simulink model "Pedal_Interpretation_exe_gr"  (Simulink 7.0)
settings: Solver=ode4  StartTime=0.0  StopTime=88  FixedStep=0.01  RelTol=1e-3
InitFcn:
  | PedalInterp_para
values from neighbouring files (symbols this model uses):
  ped_min = 5    [PedalInterp_para.m]
  T_max_Brake = 4000    [PedalInterp_para.m]
  TI = 0    [PAS_callback.m]
undefined symbols (not defined in the file or in its folder): fzgbib, m_ab_100pro, m_ab_70pro, PedalInterpretation, v_bereich
libraries: simulink x320
(part 3 of 23)

== system Pedal_Interpretation_exe_gr/Test Specification for PI/SR-PI-02.2 Acceleration pedal interpretation/v = const & phi_Acc = const ==
  InOut Bus : Inport  OutDataType=sfix(16)  OutScaling=2^0
  Bus Selector : BusSelector  OutputSignals=Inputs.v_Fzg,Inputs.signal2.phi_Acc
  Constant : Constant  OutDataType=sfix(16)  OutScaling=2^0
  Constant1 : Constant  OutDataType=sfix(16)  OutScaling=2^0
  Detect constant : Subsystem  TreatAsAtomicUnit=on  mask(Feature extraction block){RT=1}
      mask prompts: RT "Relative tolerance in %"
      mask help: Detect if the signal value is constant (using the last two signal values) allowing for a user-defined relative deviation
      mask CallbackString:
      | if or( (str2double(get_param(gcb,'RT')) < 0), (str2double(get_param(gcb,'RT')) > 100))
      |     error(['Relative tolerance value (' get_param(gcb,'RT') ') out of range. Please give a value between 0 and 100.']);
      | else
      |     set_param([gcb '/Relative tolerance/Relative Tolerance'],'Value',get_param(gcb,'RT'));
      | end
  Detect constant1 : Subsystem  TreatAsAtomicUnit=on  mask(Feature extraction block){RT=1}
      mask prompts: RT "Relative tolerance in %"
      mask help: Detect if the signal value is constant (using the last two signal values) allowing for a user-defined relative deviation
      mask CallbackString:
      | if or( (str2double(get_param(gcb,'RT')) < 0), (str2double(get_param(gcb,'RT')) > 100))
      |     error(['Relative tolerance value (' get_param(gcb,'RT') ') out of range. Please give a value between 0 and 100.']);
      | else
      |     set_param([gcb '/Relative tolerance/Relative Tolerance'],'Value',get_param(gcb,'RT'));
      | end
  PS : Subsystem  mask(Feature layer: preconditions synchronization){NoTI=2, NoTDD=0, NoTID=0, TIdel=[2  2], TDDdel=[]}
      mask prompts: NoTI "Time-independent features identifiable with or without a delay (TI)"; NoTDD "Triggered features identifiable with determinate delay or without a delay (TDD)"; NoTID "Triggered features identifiable with indeterminate delay (TID)"; TIdel "Time-independent features delays (in time steps). E.g. [0 1 0] for 3 features"; TDDdel "Triggered features delays (in time steps). E.g. [0 0] for 2 features"
      mask help: Use this block for synchronizing the precondition features. For changing the block inputs, use the parameters below. The output must be used for assertions activation.
      mask init:
      | PS_init(gcb);
      mask StyleString: popup(0|1|2|3|4|5|6|7|8|9),popup(0|1|2|3|4|5|6|7|8|9),popup(0|1|2|3|4|5|6|7|8|9),edit,edit
      mask CallbackString:
      | PSTI_callback(gcb);|PSTDD_callback(gcb);|PSTID_callback(gcb);|NoTI = str2double(get_param(gcb,'NoTI'));
      | TIdel = str2num(get_param(gcb,'TIdel'));
      | if NoTI ~= length(TIdel) && NoTI ~= 0
      |     error(['The number of delays entered (' num2str(length(TIdel)) ') does not correspond to the above specified number of time-independent features (' num2str(NoTI) ').']);
      | end|NoTDD = str2double(get_param(gcb,'NoTDD'));
      | TDDdel = str2num(get_param(gcb,'TDDdel'));
      | if NoTDD ~= length(TDDdel) && NoTDD ~= 0
      |     error(['The number of delays entered (' num2str(length(TDDdel)) ') does not correspond to the above specified number of triggered features with constant delay (' num2str(NoTDD) ').']);
      | end
  Range - Gap Relative tolerance Precond : Subsystem  mask(Range - Gap Relative Tolerance){GorR=Range, RelativeTolerance=0}
      mask prompts: GorR "Use range or gap"; RelativeTolerance "Relative Tolerance in Percent"
      mask help: Check that a signal stays inside a range or outside a gap around a reference signal. Specify the range or the gap relative to the reference signal.
      mask init: same as Pedal_Interpretation_exe_gr/Test Specification for PI/SR-PI-01.1 Brake Pedal recognition/BrakePedal == 0/Range - Gap Relative tolerance Ass
      mask StyleString: popup(Range|Gap  ),edit
      mask Display:
      | port_label('output',1,'A');
      | port_label('input',1,'Sig');
      | port_label('input',2,'Ref');
      | text(0.35,0.5,[num2str(RelativeTolerance) '%']);
      | text(0.05,0.5,helpVariable2);
  Range - Gap Relative tolerance Precond1 : Subsystem  mask(Range - Gap Relative Tolerance){GorR=Range, RelativeTolerance=0}
      mask prompts: GorR "Use range or gap"; RelativeTolerance "Relative Tolerance in Percent"
      mask help: Check that a signal stays inside a range or outside a gap around a reference signal. Specify the range or the gap relative to the reference signal.
      mask init: same as Pedal_Interpretation_exe_gr/Test Specification for PI/SR-PI-01.1 Brake Pedal recognition/BrakePedal == 0/Range - Gap Relative tolerance Ass
      mask StyleString: popup(Range|Gap  ),edit
      mask Display:
      | port_label('output',1,'A');
      | port_label('input',1,'Sig');
      | port_label('input',2,'Ref');
      | text(0.35,0.5,[num2str(RelativeTolerance) '%']);
      | text(0.05,0.5,helpVariable2);
  Activate : Outport  OutDataType=sfix(16)  OutScaling=2^0
  wires:
  InOut Bus/1 -> Bus Selector/1
  Bus Selector/1 -> Detect constant/1(Signal)  "<v_Fzg>"
  Bus Selector/2 -> Detect constant1/1(Signal)  "<phi_Acc>"
  PS/1(Precond) -> Activate/1
  Detect constant/1(Constant) -> Range - Gap Relative tolerance Precond/1(Signal)
  Constant/1 -> Range - Gap Relative tolerance Precond/2(Reference)
  Detect constant1/1(Constant) -> Range - Gap Relative tolerance Precond1/1(Signal)
  Constant1/1 -> Range - Gap Relative tolerance Precond1/2(Reference)
  Range - Gap Relative tolerance Precond/1(Activate) -> PS/1(A TI1)
  Range - Gap Relative tolerance Precond1/1(Activate) -> PS/2(A TI2)

== system Pedal_Interpretation_exe_gr/Test Specification for PI/SR-PI-02.2 Acceleration pedal interpretation/v = const & phi_Acc decreases & T_des_Drive < 0 ==
  InOut Bus : Inport  OutDataType=sfix(16)  OutScaling=2^0
  Bound Precond : Subsystem  mask(Bound){cm=<}
      mask prompts: cm "Comparison method:"
      mask help:
      | Compare a signal with a reference using the specified comparison method.
      |
      | For '==' or '~=' use "Range - Gap"
      mask init:
      | bp = get_param(gcbh,'Parent');
      | bn = get_param(gcbh,'Name');
      | set_param([bp '/' bn '/RelOp'],'Operator',get_param(gcbh,'cm'));
      mask StyleString: popup(>|>=|<=|<)
      mask Display:
      | port_label('output', 1, 'A');
      | port_label('input', 1, 'Sig');
      | port_label('input', 2, 'Ref');
      | text(0.05,0.5,get_param(get_param([get_param(gcb,'Parent') '/' get_param(gcb,'Name') '/RelOp'],'handle'),'Operator'));
  Bus Selector : BusSelector  OutputSignals=Inputs.v_Fzg,Inputs.signal2.phi_Acc,Outputs.signal1.T_des_Drive
  Constant : Constant  OutDataType=sfix(16)  OutScaling=2^0
  Constant1 : Constant  OutDataType=sfix(16)  OutScaling=2^0
  Constant2 : Constant  Value=0  OutDataType=sfix(16)  OutScaling=2^0
  Detect constant : Subsystem  TreatAsAtomicUnit=on  mask(Feature extraction block){RT=0}
      mask prompts: RT "Relative tolerance in %"
      mask help: Detect if the signal value is constant (using the last two signal values) allowing for a user-defined relative deviation
      mask CallbackString:
      | if or( (str2double(get_param(gcb,'RT')) < 0), (str2double(get_param(gcb,'RT')) > 100))
      |     error(['Relative tolerance value (' get_param(gcb,'RT') ') out of range. Please give a value between 0 and 100.']);
      | else
      |     set_param([gcb '/Relative tolerance/Relative Tolerance'],'Value',get_param(gcb,'RT'));
      | end
  Detect decrease : Subsystem  TreatAsAtomicUnit=on  mask(Detect increase){Param=0}
      mask prompts: Param "Mask Parameter 1:"
  PS : Subsystem  mask(Feature layer: preconditions synchronization){NoTI=3, NoTDD=0, NoTID=0, TIdel=[2  2  2], TDDdel=[]}
      mask prompts: NoTI "Time-independent features identifiable with or without a delay (TI)"; NoTDD "Triggered features identifiable with determinate delay or without a delay (TDD)"; NoTID "Triggered features identifiable with indeterminate delay (TID)"; TIdel "Time-independent features delays (in time steps). E.g. [0 1 0] for 3 features"; TDDdel "Triggered features delays (in time steps). E.g. [0 0] for 2 features"
      mask help: Use this block for synchronizing the precondition features. For changing the block inputs, use the parameters below. The output must be used for assertions activation.
      mask init:
      | PS_init(gcb);
      mask StyleString: popup(0|1|2|3|4|5|6|7|8|9),popup(0|1|2|3|4|5|6|7|8|9),popup(0|1|2|3|4|5|6|7|8|9),edit,edit
      mask CallbackString:
      | PSTI_callback(gcb);|PSTDD_callback(gcb);|PSTID_callback(gcb);|NoTI = str2double(get_param(gcb,'NoTI'));
      | TIdel = str2num(get_param(gcb,'TIdel'));
      | if NoTI ~= length(TIdel) && NoTI ~= 0
      |     error(['The number of delays entered (' num2str(length(TIdel)) ') does not correspond to the above specified number of time-independent features (' num2str(NoTI) ').']);
      | end|NoTDD = str2double(get_param(gcb,'NoTDD'));
      | TDDdel = str2num(get_param(gcb,'TDDdel'));
      | if NoTDD ~= length(TDDdel) && NoTDD ~= 0
      |     error(['The number of delays entered (' num2str(length(TDDdel)) ') does not correspond to the above specified number of triggered features with constant delay (' num2str(NoTDD) ').']);
      | end
  Range - Gap Relative tolerance Precond : Subsystem  mask(Range - Gap Relative Tolerance){GorR=Range, RelativeTolerance=0}
      mask prompts: GorR "Use range or gap"; RelativeTolerance "Relative Tolerance in Percent"
      mask help: Check that a signal stays inside a range or outside a gap around a reference signal. Specify the range or the gap relative to the reference signal.
      mask init: same as Pedal_Interpretation_exe_gr/Test Specification for PI/SR-PI-01.1 Brake Pedal recognition/BrakePedal == 0/Range - Gap Relative tolerance Ass
      mask StyleString: popup(Range|Gap  ),edit
      mask Display:
      | port_label('output',1,'A');
      | port_label('input',1,'Sig');
      | port_label('input',2,'Ref');
      | text(0.35,0.5,[num2str(RelativeTolerance) '%']);
      | text(0.05,0.5,helpVariable2);
  Range - Gap Relative tolerance Precond1 : Subsystem  mask(Range - Gap Relative Tolerance){GorR=Range, RelativeTolerance=0}
      mask prompts: GorR "Use range or gap"; RelativeTolerance "Relative Tolerance in Percent"
      mask help: Check that a signal stays inside a range or outside a gap around a reference signal. Specify the range or the gap relative to the reference signal.
      mask init: same as Pedal_Interpretation_exe_gr/Test Specification for PI/SR-PI-01.1 Brake Pedal recognition/BrakePedal == 0/Range - Gap Relative tolerance Ass
      mask StyleString: popup(Range|Gap  ),edit
      mask Display:
      | port_label('output',1,'A');
      | port_label('input',1,'Sig');
      | port_label('input',2,'Ref');
      | text(0.35,0.5,[num2str(RelativeTolerance) '%']);
      | text(0.05,0.5,helpVariable2);
  Scope1 : Scope  NumInputPorts=4
      settings: YMin=-5~-5~-5~-5  YMax=5~5~5~5  SaveName=ScopeData10  MaxDataPoints=11115000
  Activate : Outport  OutDataType=sfix(16)  OutScaling=2^0
  wires:
  PS/1(Precond) -> Activate/1
  InOut Bus/1 -> Bus Selector/1
  Bus Selector/1 -> Detect constant/1(Signal)  "<v_Fzg>"
  Bus Selector/2 -> Detect decrease/1(Signal)  "<phi_Acc>"
  Constant/1 -> Range - Gap Relative tolerance Precond/2(Reference)
  Constant1/1 -> Range - Gap Relative tolerance Precond1/2(Reference)
  Range - Gap Relative tolerance Precond/1(Verdict) -> PS/1(A TI1), Scope1/1
  Range - Gap Relative tolerance Precond1/1(Verdict) -> PS/2(A TI2), Scope1/2
  Detect constant/1(Constant) -> Range - Gap Relative tolerance Precond/1(Signal)
  Detect decrease/1(Decrease) -> Range - Gap Relative tolerance Precond1/1(Signal)
  Bus Selector/3 -> Bound Precond/1(Signal)  "<T_des_Drive>"
  Constant2/1 -> Bound Precond/2(Reference)
  Bound Precond/1(Activate) -> PS/3(A TI3)

== system Pedal_Interpretation_exe_gr/Test Specification for PI/SR-PI-02.2 Acceleration pedal interpretation/v = const & phi_Acc decreases & T_des_Drive >= 0 ==
  InOut Bus : Inport  OutDataType=sfix(16)  OutScaling=2^0
  Bound Precond : Subsystem  mask(Bound){cm=>=}
      mask prompts: cm "Comparison method:"
      mask help:
      | Compare a signal with a reference using the specified comparison method.
      |
      | For '==' or '~=' use "Range - Gap"
      mask init:
      | bp = get_param(gcbh,'Parent');
      | bn = get_param(gcbh,'Name');
      | set_param([bp '/' bn '/RelOp'],'Operator',get_param(gcbh,'cm'));
      mask StyleString: popup(>|>=|<=|<)
      mask Display:
      | port_label('output', 1, 'A');
      | port_label('input', 1, 'Sig');
      | port_label('input', 2, 'Ref');
      | text(0.05,0.5,get_param(get_param([get_param(gcb,'Parent') '/' get_param(gcb,'Name') '/RelOp'],'handle'),'Operator'));
  Bus Selector : BusSelector  OutputSignals=Inputs.v_Fzg,Inputs.signal2.phi_Acc,Outputs.signal1.T_des_Drive
  Constant : Constant  OutDataType=sfix(16)  OutScaling=2^0
  Constant1 : Constant  OutDataType=sfix(16)  OutScaling=2^0
  Constant2 : Constant  Value=0  OutDataType=sfix(16)  OutScaling=2^0
  Detect constant : Subsystem  TreatAsAtomicUnit=on  mask(Feature extraction block){RT=0}
      mask prompts: RT "Relative tolerance in %"
      mask help: Detect if the signal value is constant (using the last two signal values) allowing for a user-defined relative deviation
      mask CallbackString:
      | if or( (str2double(get_param(gcb,'RT')) < 0), (str2double(get_param(gcb,'RT')) > 100))
      |     error(['Relative tolerance value (' get_param(gcb,'RT') ') out of range. Please give a value between 0 and 100.']);
      | else
      |     set_param([gcb '/Relative tolerance/Relative Tolerance'],'Value',get_param(gcb,'RT'));
      | end
  Detect decrease : Subsystem  TreatAsAtomicUnit=on  mask(Detect increase){Param=0}
      mask prompts: Param "Mask Parameter 1:"
  PS : Subsystem  mask(Feature layer: preconditions synchronization){NoTI=3, NoTDD=0, NoTID=0, TIdel=[2  2  2], TDDdel=[]}
      mask prompts: NoTI "Time-independent features identifiable with or without a delay (TI)"; NoTDD "Triggered features identifiable with determinate delay or without a delay (TDD)"; NoTID "Triggered features identifiable with indeterminate delay (TID)"; TIdel "Time-independent features delays (in time steps). E.g. [0 1 0] for 3 features"; TDDdel "Triggered features delays (in time steps). E.g. [0 0] for 2 features"
      mask help: Use this block for synchronizing the precondition features. For changing the block inputs, use the parameters below. The output must be used for assertions activation.
      mask init:
      | PS_init(gcb);
      mask StyleString: popup(0|1|2|3|4|5|6|7|8|9),popup(0|1|2|3|4|5|6|7|8|9),popup(0|1|2|3|4|5|6|7|8|9),edit,edit
      mask CallbackString:
      | PSTI_callback(gcb);|PSTDD_callback(gcb);|PSTID_callback(gcb);|NoTI = str2double(get_param(gcb,'NoTI'));
      | TIdel = str2num(get_param(gcb,'TIdel'));
      | if NoTI ~= length(TIdel) && NoTI ~= 0
      |     error(['The number of delays entered (' num2str(length(TIdel)) ') does not correspond to the above specified number of time-independent features (' num2str(NoTI) ').']);
      | end|NoTDD = str2double(get_param(gcb,'NoTDD'));
      | TDDdel = str2num(get_param(gcb,'TDDdel'));
      | if NoTDD ~= length(TDDdel) && NoTDD ~= 0
      |     error(['The number of delays entered (' num2str(length(TDDdel)) ') does not correspond to the above specified number of triggered features with constant delay (' num2str(NoTDD) ').']);
      | end
  Range - Gap Relative tolerance Precond : Subsystem  mask(Range - Gap Relative Tolerance){GorR=Range, RelativeTolerance=0}
      mask prompts: GorR "Use range or gap"; RelativeTolerance "Relative Tolerance in Percent"
      mask help: Check that a signal stays inside a range or outside a gap around a reference signal. Specify the range or the gap relative to the reference signal.
      mask init: same as Pedal_Interpretation_exe_gr/Test Specification for PI/SR-PI-01.1 Brake Pedal recognition/BrakePedal == 0/Range - Gap Relative tolerance Ass
      mask StyleString: popup(Range|Gap  ),edit
      mask Display:
      | port_label('output',1,'A');
      | port_label('input',1,'Sig');
      | port_label('input',2,'Ref');
      | text(0.35,0.5,[num2str(RelativeTolerance) '%']);
      | text(0.05,0.5,helpVariable2);
  Range - Gap Relative tolerance Precond1 : Subsystem  mask(Range - Gap Relative Tolerance){GorR=Range, RelativeTolerance=0}
      mask prompts: GorR "Use range or gap"; RelativeTolerance "Relative Tolerance in Percent"
      mask help: Check that a signal stays inside a range or outside a gap around a reference signal. Specify the range or the gap relative to the reference signal.
      mask init: same as Pedal_Interpretation_exe_gr/Test Specification for PI/SR-PI-01.1 Brake Pedal recognition/BrakePedal == 0/Range - Gap Relative tolerance Ass
      mask StyleString: popup(Range|Gap  ),edit
      mask Display:
      | port_label('output',1,'A');
      | port_label('input',1,'Sig');
      | port_label('input',2,'Ref');
      | text(0.35,0.5,[num2str(RelativeTolerance) '%']);
      | text(0.05,0.5,helpVariable2);
  Scope1 : Scope  NumInputPorts=4
      settings: YMin=-5~-5~-5~-5  YMax=5~5~5~5  SaveName=ScopeData10  MaxDataPoints=11115000
  Activate : Outport  OutDataType=sfix(16)  OutScaling=2^0
  wires:
  PS/1(Precond) -> Activate/1
  InOut Bus/1 -> Bus Selector/1
  Bus Selector/1 -> Detect constant/1(Signal)  "<v_Fzg>"
  Bus Selector/2 -> Detect decrease/1(Signal)  "<phi_Acc>"
  Constant/1 -> Range - Gap Relative tolerance Precond/2(Reference)
  Constant1/1 -> Range - Gap Relative tolerance Precond1/2(Reference)
  Range - Gap Relative tolerance Precond/1(Verdict) -> PS/1(A TI1), Scope1/1
  Range - Gap Relative tolerance Precond1/1(Verdict) -> PS/2(A TI2), Scope1/2
  Detect constant/1(Constant) -> Range - Gap Relative tolerance Precond/1(Signal)
  Detect decrease/1(Decrease) -> Range - Gap Relative tolerance Precond1/1(Signal)
  Bus Selector/3 -> Bound Precond/1(Signal)  "<T_des_Drive>"
  Constant2/1 -> Bound Precond/2(Reference)
  Bound Precond/1(Activate) -> PS/3(A TI3)

== system Pedal_Interpretation_exe_gr/Test Specification for PI/SR-PI-02.2 Acceleration pedal interpretation/v = const & phi_Acc increases & T_des_Drive < 0 ==
  InOut Bus : Inport  OutDataType=sfix(16)  OutScaling=2^0
  Bound Precond : Subsystem  mask(Bound){cm=<}
      mask prompts: cm "Comparison method:"
      mask help:
      | Compare a signal with a reference using the specified comparison method.
      |
      | For '==' or '~=' use "Range - Gap"
      mask init:
      | bp = get_param(gcbh,'Parent');
      | bn = get_param(gcbh,'Name');
      | set_param([bp '/' bn '/RelOp'],'Operator',get_param(gcbh,'cm'));
      mask StyleString: popup(>|>=|<=|<)
      mask Display:
      | port_label('output', 1, 'A');
      | port_label('input', 1, 'Sig');
      | port_label('input', 2, 'Ref');
      | text(0.05,0.5,get_param(get_param([get_param(gcb,'Parent') '/' get_param(gcb,'Name') '/RelOp'],'handle'),'Operator'));
  Bus Selector : BusSelector  OutputSignals=Inputs.v_Fzg,Inputs.signal2.phi_Acc,Outputs.signal1.T_des_Drive
  Constant : Constant  OutDataType=sfix(16)  OutScaling=2^0
  Constant1 : Constant  OutDataType=sfix(16)  OutScaling=2^0
  Constant2 : Constant  Value=0  OutDataType=sfix(16)  OutScaling=2^0
  Detect constant : Subsystem  TreatAsAtomicUnit=on  mask(Feature extraction block){RT=0}
      mask prompts: RT "Relative tolerance in %"
      mask help: Detect if the signal value is constant (using the last two signal values) allowing for a user-defined relative deviation
      mask CallbackString:
      | if or( (str2double(get_param(gcb,'RT')) < 0), (str2double(get_param(gcb,'RT')) > 100))
      |     error(['Relative tolerance value (' get_param(gcb,'RT') ') out of range. Please give a value between 0 and 100.']);
      | else
      |     set_param([gcb '/Relative tolerance/Relative Tolerance'],'Value',get_param(gcb,'RT'));
      | end
  Detect increase : Subsystem  TreatAsAtomicUnit=on  mask(Detect increase){Param=0}
      mask prompts: Param "Mask Parameter 1:"
  PS : Subsystem  mask(Feature layer: preconditions synchronization){NoTI=3, NoTDD=0, NoTID=0, TIdel=[2  2  0], TDDdel=[]}
      mask prompts: NoTI "Time-independent features identifiable with or without a delay (TI)"; NoTDD "Triggered features identifiable with determinate delay or without a delay (TDD)"; NoTID "Triggered features identifiable with indeterminate delay (TID)"; TIdel "Time-independent features delays (in time steps). E.g. [0 1 0] for 3 features"; TDDdel "Triggered features delays (in time steps). E.g. [0 0] for 2 features"
      mask help: Use this block for synchronizing the precondition features. For changing the block inputs, use the parameters below. The output must be used for assertions activation.
      mask init:
      | PS_init(gcb);
      mask StyleString: popup(0|1|2|3|4|5|6|7|8|9),popup(0|1|2|3|4|5|6|7|8|9),popup(0|1|2|3|4|5|6|7|8|9),edit,edit
      mask CallbackString:
      | PSTI_callback(gcb);|PSTDD_callback(gcb);|PSTID_callback(gcb);|NoTI = str2double(get_param(gcb,'NoTI'));
      | TIdel = str2num(get_param(gcb,'TIdel'));
      | if NoTI ~= length(TIdel) && NoTI ~= 0
      |     error(['The number of delays entered (' num2str(length(TIdel)) ') does not correspond to the above specified number of time-independent features (' num2str(NoTI) ').']);
      | end|NoTDD = str2double(get_param(gcb,'NoTDD'));
      | TDDdel = str2num(get_param(gcb,'TDDdel'));
      | if NoTDD ~= length(TDDdel) && NoTDD ~= 0
      |     error(['The number of delays entered (' num2str(length(TDDdel)) ') does not correspond to the above specified number of triggered features with constant delay (' num2str(NoTDD) ').']);
      | end
  Range - Gap Relative tolerance Precond : Subsystem  mask(Range - Gap Relative Tolerance){GorR=Range, RelativeTolerance=0}
      mask prompts: GorR "Use range or gap"; RelativeTolerance "Relative Tolerance in Percent"
      mask help: Check that a signal stays inside a range or outside a gap around a reference signal. Specify the range or the gap relative to the reference signal.
      mask init: same as Pedal_Interpretation_exe_gr/Test Specification for PI/SR-PI-01.1 Brake Pedal recognition/BrakePedal == 0/Range - Gap Relative tolerance Ass
      mask StyleString: popup(Range|Gap  ),edit
      mask Display:
      | port_label('output',1,'A');
      | port_label('input',1,'Sig');
      | port_label('input',2,'Ref');
      | text(0.35,0.5,[num2str(RelativeTolerance) '%']);
      | text(0.05,0.5,helpVariable2);
  Range - Gap Relative tolerance Precond1 : Subsystem  mask(Range - Gap Relative Tolerance){GorR=Range, RelativeTolerance=0}
      mask prompts: GorR "Use range or gap"; RelativeTolerance "Relative Tolerance in Percent"
      mask help: Check that a signal stays inside a range or outside a gap around a reference signal. Specify the range or the gap relative to the reference signal.
      mask init: same as Pedal_Interpretation_exe_gr/Test Specification for PI/SR-PI-01.1 Brake Pedal recognition/BrakePedal == 0/Range - Gap Relative tolerance Ass
      mask StyleString: popup(Range|Gap  ),edit
      mask Display:
      | port_label('output',1,'A');
      | port_label('input',1,'Sig');
      | port_label('input',2,'Ref');
      | text(0.35,0.5,[num2str(RelativeTolerance) '%']);
      | text(0.05,0.5,helpVariable2);
  Activate : Outport  OutDataType=sfix(16)  OutScaling=2^0
  wires:
  InOut Bus/1 -> Bus Selector/1
  Bus Selector/2 -> Detect increase/1(Signal)  "<phi_Acc>"
  Bus Selector/1 -> Detect constant/1(Signal)  "<v_Fzg>"
  PS/1(Precond) -> Activate/1
  Detect constant/1(Constant) -> Range - Gap Relative tolerance Precond/1(Signal)
  Range - Gap Relative tolerance Precond/1(Activate) -> PS/1(A TI1)
  Constant/1 -> Range - Gap Relative tolerance Precond/2(Reference)
  Detect increase/1(Increase) -> Range - Gap Relative tolerance Precond1/1(Signal)
  Range - Gap Relative tolerance Precond1/1(Activate) -> PS/2(A TI2)
  Constant1/1 -> Range - Gap Relative tolerance Precond1/2(Reference)
  Bus Selector/3 -> Bound Precond/1(Signal)  "<T_des_Drive>"
  Constant2/1 -> Bound Precond/2(Reference)
  Bound Precond/1(Activate) -> PS/3(A TI3)

== system Pedal_Interpretation_exe_gr/Test Specification for PI/SR-PI-02.2 Acceleration pedal interpretation/v = const & phi_Acc increases & T_des_Drive >= 0 ==
  InOut Bus : Inport  OutDataType=sfix(16)  OutScaling=2^0
  "  " : Subsystem  mask(Range - Gap Relative Tolerance){GorR=Range, RelativeTolerance=0}
      mask prompts: GorR "Use range or gap"; RelativeTolerance "Relative Tolerance in Percent"
      mask help: Check that a signal stays inside a range or outside a gap around a reference signal. Specify the range or the gap relative to the reference signal.
      mask init: same as Pedal_Interpretation_exe_gr/Test Specification for PI/SR-PI-01.1 Brake Pedal recognition/BrakePedal == 0/Range - Gap Relative tolerance Ass
      mask StyleString: popup(Range|Gap  ),edit
      mask Display:
      | port_label('output',1,'A');
      | port_label('input',1,'Sig');
      | port_label('input',2,'Ref');
      | text(0.35,0.5,[num2str(RelativeTolerance) '%']);
      | text(0.05,0.5,helpVariable2);
  "    " : Subsystem  mask(Range - Gap Relative Tolerance){GorR=Range, RelativeTolerance=0}
      mask prompts: GorR "Use range or gap"; RelativeTolerance "Relative Tolerance in Percent"
      mask help: Check that a signal stays inside a range or outside a gap around a reference signal. Specify the range or the gap relative to the reference signal.
      mask init: same as Pedal_Interpretation_exe_gr/Test Specification for PI/SR-PI-01.1 Brake Pedal recognition/BrakePedal == 0/Range - Gap Relative tolerance Ass
      mask StyleString: popup(Range|Gap  ),edit
      mask Display:
      | port_label('output',1,'A');
      | port_label('input',1,'Sig');
      | port_label('input',2,'Ref');
      | text(0.35,0.5,[num2str(RelativeTolerance) '%']);
      | text(0.05,0.5,helpVariable2);
  "        " : Subsystem  mask(Bound){cm=>=}
      mask prompts: cm "Comparison method:"
      mask help:
      | Compare a signal with a reference using the specified comparison method.
      |
      | For '==' or '~=' use "Range - Gap"
      mask init:
      | bp = get_param(gcbh,'Parent');
      | bn = get_param(gcbh,'Name');
      | set_param([bp '/' bn '/RelOp'],'Operator',get_param(gcbh,'cm'));
      mask StyleString: popup(>|>=|<=|<)
      mask Display:
      | port_label('output', 1, 'A');
      | port_label('input', 1, 'Sig');
      | port_label('input', 2, 'Ref');
      | text(0.05,0.5,get_param(get_param([get_param(gcb,'Parent') '/' get_param(gcb,'Name') '/RelOp'],'handle'),'Operator'));
  Bus Selector : BusSelector  OutputSignals=Inputs.v_Fzg,Inputs.signal2.phi_Acc,Outputs.signal1.T_des_Drive
  Detect constant : Subsystem  TreatAsAtomicUnit=on  mask(Feature extraction block){RT=0}
      mask prompts: RT "Relative tolerance in %"
      mask help: Detect if the signal value is constant (using the last two signal values) allowing for a user-defined relative deviation
      mask CallbackString:
      | if or( (str2double(get_param(gcb,'RT')) < 0), (str2double(get_param(gcb,'RT')) > 100))
      |     error(['Relative tolerance value (' get_param(gcb,'RT') ') out of range. Please give a value between 0 and 100.']);
      | else
      |     set_param([gcb '/Relative tolerance/Relative Tolerance'],'Value',get_param(gcb,'RT'));
      | end
  Detect increase : Subsystem  TreatAsAtomicUnit=on  mask(Detect increase){Param=0}
      mask prompts: Param "Mask Parameter 1:"
  PS : Subsystem  mask(Feature layer: preconditions synchronization){NoTI=3, NoTDD=0, NoTID=0, TIdel=[2  2  0], TDDdel=[]}
      mask prompts: NoTI "Time-independent features identifiable with or without a delay (TI)"; NoTDD "Triggered features identifiable with determinate delay or without a delay (TDD)"; NoTID "Triggered features identifiable with indeterminate delay (TID)"; TIdel "Time-independent features delays (in time steps). E.g. [0 1 0] for 3 features"; TDDdel "Triggered features delays (in time steps). E.g. [0 0] for 2 features"
      mask help: Use this block for synchronizing the precondition features. For changing the block inputs, use the parameters below. The output must be used for assertions activation.
      mask init:
      | PS_init(gcb);
      mask StyleString: popup(0|1|2|3|4|5|6|7|8|9),popup(0|1|2|3|4|5|6|7|8|9),popup(0|1|2|3|4|5|6|7|8|9),edit,edit
      mask CallbackString:
      | PSTI_callback(gcb);|PSTDD_callback(gcb);|PSTID_callback(gcb);|NoTI = str2double(get_param(gcb,'NoTI'));
      | TIdel = str2num(get_param(gcb,'TIdel'));
      | if NoTI ~= length(TIdel) && NoTI ~= 0
      |     error(['The number of delays entered (' num2str(length(TIdel)) ') does not correspond to the above specified number of time-independent features (' num2str(NoTI) ').']);
      | end|NoTDD = str2double(get_param(gcb,'NoTDD'));
      | TDDdel = str2num(get_param(gcb,'TDDdel'));
      | if NoTDD ~= length(TDDdel) && NoTDD ~= 0
      |     error(['The number of delays entered (' num2str(length(TDDdel)) ') does not correspond to the above specified number of triggered features with constant delay (' num2str(NoTDD) ').']);
      | end
  Ref : Constant  Value=0  OutDataType=sfix(16)  OutScaling=2^0
  true : Constant  OutDataType=sfix(16)  OutScaling=2^0
  "true " : Constant  OutDataType=sfix(16)  OutScaling=2^0
  Activate : Outport  OutDataType=sfix(16)  OutScaling=2^0
  wires:
  InOut Bus/1 -> Bus Selector/1
  Bus Selector/2 -> Detect increase/1(Signal)  "<phi_Acc>"
  Bus Selector/1 -> Detect constant/1(Signal)  "<v_Fzg>"
  PS/1(Precond) -> Activate/1
  Detect constant/1(Constant) -> "  "/1(Signal)
  "  "/1(Activate) -> PS/1(A TI1)
  true/1 -> "  "/2(Reference)
  Detect increase/1(Increase) -> "    "/1(Signal)
  "    "/1(Activate) -> PS/2(A TI2)
  "true "/1 -> "    "/2(Reference)
  Bus Selector/3 -> "        "/1(Signal)  "<T_des_Drive>"
  Ref/1 -> "        "/2(Reference)
  "        "/1(Activate) -> PS/3(A TI3)

== system Pedal_Interpretation_exe_gr/Test Specification for PI/SR-PI-02.2 Acceleration pedal interpretation/v increases & phi_Acc = const & T_des_Drive >= 0 ==
  InOut Bus : Inport  OutDataType=sfix(16)  OutScaling=2^0
  Bound Precond : Subsystem  mask(Bound){cm=>=}
      mask prompts: cm "Comparison method:"
      mask help:
      | Compare a signal with a reference using the specified comparison method.
      |
      | For '==' or '~=' use "Range - Gap"
      mask init:
      | bp = get_param(gcbh,'Parent');
      | bn = get_param(gcbh,'Name');
      | set_param([bp '/' bn '/RelOp'],'Operator',get_param(gcbh,'cm'));
      mask StyleString: popup(>|>=|<=|<)
      mask Display:
      | port_label('output', 1, 'A');
      | port_label('input', 1, 'Sig');
      | port_label('input', 2, 'Ref');
      | text(0.05,0.5,get_param(get_param([get_param(gcb,'Parent') '/' get_param(gcb,'Name') '/RelOp'],'handle'),'Operator'));
  Bus Selector : BusSelector  OutputSignals=Inputs.v_Fzg,Inputs.signal2.phi_Acc,Outputs.signal1.T_des_Drive
  Constant : Constant  Value=0  OutDataType=sfix(16)  OutScaling=2^0
  Constant1 : Constant  OutDataType=sfix(16)  OutScaling=2^0
  Constant2 : Constant  OutDataType=sfix(16)  OutScaling=2^0
  Detect constant : Subsystem  TreatAsAtomicUnit=on  mask(Feature extraction block){RT=0}
      mask prompts: RT "Relative tolerance in %"
      mask help: Detect if the signal value is constant (using the last two signal values) allowing for a user-defined relative deviation
      mask CallbackString:
      | if or( (str2double(get_param(gcb,'RT')) < 0), (str2double(get_param(gcb,'RT')) > 100))
      |     error(['Relative tolerance value (' get_param(gcb,'RT') ') out of range. Please give a value between 0 and 100.']);
      | else
      |     set_param([gcb '/Relative tolerance/Relative Tolerance'],'Value',get_param(gcb,'RT'));
      | end
  Detect increase : Subsystem  TreatAsAtomicUnit=on  mask(Detect increase){Param=0}
      mask prompts: Param "Mask Parameter 1:"
  PS : Subsystem  mask(Feature layer: preconditions synchronization){NoTI=3, NoTDD=0, NoTID=0, TIdel=[2  2  0], TDDdel=[]}
      mask prompts: NoTI "Time-independent features identifiable with or without a delay (TI)"; NoTDD "Triggered features identifiable with determinate delay or without a delay (TDD)"; NoTID "Triggered features identifiable with indeterminate delay (TID)"; TIdel "Time-independent features delays (in time steps). E.g. [0 1 0] for 3 features"; TDDdel "Triggered features delays (in time steps). E.g. [0 0] for 2 features"
      mask help: Use this block for synchronizing the precondition features. For changing the block inputs, use the parameters below. The output must be used for assertions activation.
      mask init:
      | PS_init(gcb);
      mask StyleString: popup(0|1|2|3|4|5|6|7|8|9),popup(0|1|2|3|4|5|6|7|8|9),popup(0|1|2|3|4|5|6|7|8|9),edit,edit
      mask CallbackString:
      | PSTI_callback(gcb);|PSTDD_callback(gcb);|PSTID_callback(gcb);|NoTI = str2double(get_param(gcb,'NoTI'));
      | TIdel = str2num(get_param(gcb,'TIdel'));
      | if NoTI ~= length(TIdel) && NoTI ~= 0
      |     error(['The number of delays entered (' num2str(length(TIdel)) ') does not correspond to the above specified number of time-independent features (' num2str(NoTI) ').']);
      | end|NoTDD = str2double(get_param(gcb,'NoTDD'));
      | TDDdel = str2num(get_param(gcb,'TDDdel'));
      | if NoTDD ~= length(TDDdel) && NoTDD ~= 0
      |     error(['The number of delays entered (' num2str(length(TDDdel)) ') does not correspond to the above specified number of triggered features with constant delay (' num2str(NoTDD) ').']);
      | end
  Range - Gap Relative tolerance Precond : Subsystem  mask(Range - Gap Relative Tolerance){GorR=Range, RelativeTolerance=0}
      mask prompts: GorR "Use range or gap"; RelativeTolerance "Relative Tolerance in Percent"
      mask help: Check that a signal stays inside a range or outside a gap around a reference signal. Specify the range or the gap relative to the reference signal.
      mask init: same as Pedal_Interpretation_exe_gr/Test Specification for PI/SR-PI-01.1 Brake Pedal recognition/BrakePedal == 0/Range - Gap Relative tolerance Ass
      mask StyleString: popup(Range|Gap  ),edit
      mask Display:
      | port_label('output',1,'A');
      | port_label('input',1,'Sig');
      | port_label('input',2,'Ref');
      | text(0.35,0.5,[num2str(RelativeTolerance) '%']);
      | text(0.05,0.5,helpVariable2);
  Range - Gap Relative tolerance Precond1 : Subsystem  mask(Range - Gap Relative Tolerance){GorR=Range, RelativeTolerance=0}
      mask prompts: GorR "Use range or gap"; RelativeTolerance "Relative Tolerance in Percent"
      mask help: Check that a signal stays inside a range or outside a gap around a reference signal. Specify the range or the gap relative to the reference signal.
      mask init: same as Pedal_Interpretation_exe_gr/Test Specification for PI/SR-PI-01.1 Brake Pedal recognition/BrakePedal == 0/Range - Gap Relative tolerance Ass
      mask StyleString: popup(Range|Gap  ),edit
      mask Display:
      | port_label('output',1,'A');
      | port_label('input',1,'Sig');
      | port_label('input',2,'Ref');
      | text(0.35,0.5,[num2str(RelativeTolerance) '%']);
      | text(0.05,0.5,helpVariable2);
  Scope1 : Scope  NumInputPorts=4
      settings: TimeRange=140  YMin=-1~-1~-5~-1  YMax=2~2~5~2  MaxDataPoints=11115000
  Activate : Outport  OutDataType=sfix(16)  OutScaling=2^0
  wires:
  PS/1(Precond) -> Activate/1
  Bus Selector/1 -> Detect increase/1(Signal)  "<v_Fzg>"
  InOut Bus/1 -> Bus Selector/1
  Bus Selector/3 -> Bound Precond/1(Signal)  "<T_des_Drive>"
  Constant/1 -> Bound Precond/2(Reference)
  Bus Selector/2 -> Detect constant/1(Signal)  "<phi_Acc>"
  Range - Gap Relative tolerance Precond/1(Activate) -> PS/1(A TI1), Scope1/1
  Range - Gap Relative tolerance Precond1/1(Activate) -> PS/2(A TI2), Scope1/2
  Bound Precond/1(Activate) -> PS/3(A TI3)
  Detect constant/1(Constant) -> Range - Gap Relative tolerance Precond/1(Signal)
  Constant1/1 -> Range - Gap Relative tolerance Precond/2(Reference)
  Detect increase/1(Increase) -> Range - Gap Relative tolerance Precond1/1(Signal)
  Constant2/1 -> Range - Gap Relative tolerance Precond1/2(Reference)

== system Pedal_Interpretation_exe_gr/Test Data for PI/SR-PI-01.1 Brake Pedal recognition/phi_Brake < ped_min/Generate decrease 2 ==
  Generate  limited decrease for partition1 variant1 1 : Subsystem  mask(Feature generation){X0=5, XF=4.5, T=2}
      mask prompts: X0 "Initial output:"; XF "Final output:"; T "Duration"
      mask help: Output a decreasing ramp signal limited from bottom and top, starting at the specified time.
      mask Display:
      | plot([1:10],[4,4,4,4,4,1,1,1,1,1])
      | plot([1:10],[4,4,4,1,1,1,1,1,1,1])
      | plot([1:10],[4,1,1,1,1,1,1,1,1,1])
      | plot([1:10],[4,4,4,4,4,1,1,1,1,1])
      | plot([1:10],[4,4,4,4,4,4,4,1,1,1])
      | plot([1:10],[4,4,4,4,4,4,4,4,4,1])
      | plot([1:10],[4,4,4,4,4,4,4,4,4,4])
      | color('white');
      | plot([1:10],[1,1,1,1,1,1,1,1,1,1])
      | color('black');
      | plot([1,1.5],[1,1])
      | plot([2.5,3.5],[1,1])
      | plot([4.5,5.5],[1,1])
      | plot([6.5,7.5],[1,1])
      | plot([8.5,9.5],[1,1])
      | color('white');
      | plot([1,1.5],[4,4])
      | plot([2.5,3.5],[4,4])
      | plot([4.5,5.5],[4,4])
      | plot([6.5,7.5],[4,4])
      | plot([8.5,9.5],[4,4])
  Generate  limited decrease for partition1 variant2 1 : Subsystem  mask(Feature generation){X0=0.5, XF=0, T=2}
      mask prompts: X0 "Initial output:"; XF "Final output:"; T "Duration"
      mask help: Output a decreasing ramp signal limited from bottom and top, starting at the specified time.
      mask Display:
      | plot([1:10],[4,4,4,4,4,1,1,1,1,1])
      | plot([1:10],[4,4,4,1,1,1,1,1,1,1])
      | plot([1:10],[4,1,1,1,1,1,1,1,1,1])
      | plot([1:10],[4,4,4,4,4,1,1,1,1,1])
      | plot([1:10],[4,4,4,4,4,4,4,1,1,1])
      | plot([1:10],[4,4,4,4,4,4,4,4,4,1])
      | plot([1:10],[4,4,4,4,4,4,4,4,4,4])
      | color('white');
      | plot([1:10],[1,1,1,1,1,1,1,1,1,1])
      | color('black');
      | plot([1,1.5],[1,1])
      | plot([2.5,3.5],[1,1])
      | plot([4.5,5.5],[1,1])
      | plot([6.5,7.5],[1,1])
      | plot([8.5,9.5],[1,1])
      | color('white');
      | plot([1,1.5],[4,4])
      | plot([2.5,3.5],[4,4])
      | plot([4.5,5.5],[4,4])
      | plot([6.5,7.5],[4,4])
      | plot([8.5,9.5],[4,4])
  TestDataVariants Sequence : Subsystem
  switch : MultiPortSwitch  Inputs=2  OutDataType=sfix(16)  OutScaling=2^0
  phi_Brake : Outport  OutDataType=sfix(16)  OutScaling=2^0
  wires:
  switch/1 -> phi_Brake/1
  Generate  limited decrease for partition1 variant2 1/1(Out1) -> switch/3
  Generate  limited decrease for partition1 variant1 1/1(Out1) -> switch/2
  TestDataVariants Sequence/1(Out1) -> switch/1

== system Pedal_Interpretation_exe_gr/Test Data for PI/SR-PI-01.1 Brake Pedal recognition/phi_Brake >= ped_min/Generate increase 2 ==
  Generate  limited increase for partition1 variant1 1 : Subsystem  mask(Feature generation){X0=5, XF=14.5, T=2}
      mask prompts: X0 "Initial output:"; XF "Final output:"; T "Duration:"
      mask help: Output a ramp signal limited from bottom and top, starting at the specified time.
      mask Display:
      | plot([1:10],[1,1,1,1,1,4,4,4,4,4])
      | plot([1:10],[1,4,4,4,4,4,4,4,4,4])
      | plot([1:10],[1,1,1,4,4,4,4,4,4,4])
      | plot([1:10],[1,1,1,1,1,4,4,4,4,4])
      | plot([1:10],[1,1,1,1,1,1,1,4,4,4])
      | plot([1:10],[1,1,1,1,1,1,1,1,1,4])
      | plot([5:10],[1,1,1,1,1,1])
      | color('white');
      | plot([1:10],[4,4,4,4,4,4,4,4,4,4])
      | color('white');
      | plot([1,1.5],[1,1])
      | plot([2.5,3.5],[1,1])
      | plot([4.5,5.5],[1,1])
      | plot([6.5,7.5],[1,1])
      | plot([8.5,9.5],[1,1])
      | color('black');
      | plot([1,1.5],[4,4])
      | plot([2.5,3.5],[4,4])
      | plot([4.5,5.5],[4,4])
      | plot([6.5,7.5],[4,4])
      | plot([8.5,9.5],[4,4])
  Generate  limited increase for partition1 variant2 1 : Subsystem  mask(Feature generation){X0=90.5, XF=100, T=2}
      mask prompts: X0 "Initial output:"; XF "Final output:"; T "Duration:"
      mask help: Output a ramp signal limited from bottom and top, starting at the specified time.
      mask Display:
      | plot([1:10],[1,1,1,1,1,4,4,4,4,4])
      | plot([1:10],[1,4,4,4,4,4,4,4,4,4])
      | plot([1:10],[1,1,1,4,4,4,4,4,4,4])
      | plot([1:10],[1,1,1,1,1,4,4,4,4,4])
      | plot([1:10],[1,1,1,1,1,1,1,4,4,4])
      | plot([1:10],[1,1,1,1,1,1,1,1,1,4])
      | plot([5:10],[1,1,1,1,1,1])
      | color('white');
      | plot([1:10],[4,4,4,4,4,4,4,4,4,4])
      | color('white');
      | plot([1,1.5],[1,1])
      | plot([2.5,3.5],[1,1])
      | plot([4.5,5.5],[1,1])
      | plot([6.5,7.5],[1,1])
      | plot([8.5,9.5],[1,1])
      | color('black');
      | plot([1,1.5],[4,4])
      | plot([2.5,3.5],[4,4])
      | plot([4.5,5.5],[4,4])
      | plot([6.5,7.5],[4,4])
      | plot([8.5,9.5],[4,4])
  TestDataVariants Sequence : Subsystem
  switch : MultiPortSwitch  Inputs=2  OutDataType=sfix(16)  OutScaling=2^0
  phi_Brake : Outport  OutDataType=sfix(16)  OutScaling=2^0
  wires:
  switch/1 -> phi_Brake/1
  Generate  limited increase for partition1 variant2 1/1(Out1) -> switch/3
  Generate  limited increase for partition1 variant1 1/1(Out1) -> switch/2
  TestDataVariants Sequence/1(Out1) -> switch/1

== system Pedal_Interpretation_exe_gr/Test Data for PI/SR-PI-01.3 Acceleration Pedal recognition/phi_Acc < ped_min/Generate decrease 2 ==
  Generate  limited decrease for partition1 variant1 1 : Subsystem  mask(Feature generation){X0=5, XF=4.5, T=2}
      mask prompts: X0 "Initial output:"; XF "Final output:"; T "Duration"
      mask help: Output a decreasing ramp signal limited from bottom and top, starting at the specified time.
      mask Display:
      | plot([1:10],[4,4,4,4,4,1,1,1,1,1])
      | plot([1:10],[4,4,4,1,1,1,1,1,1,1])
      | plot([1:10],[4,1,1,1,1,1,1,1,1,1])
      | plot([1:10],[4,4,4,4,4,1,1,1,1,1])
      | plot([1:10],[4,4,4,4,4,4,4,1,1,1])
      | plot([1:10],[4,4,4,4,4,4,4,4,4,1])
      | plot([1:10],[4,4,4,4,4,4,4,4,4,4])
      | color('white');
      | plot([1:10],[1,1,1,1,1,1,1,1,1,1])
      | color('black');
      | plot([1,1.5],[1,1])
      | plot([2.5,3.5],[1,1])
      | plot([4.5,5.5],[1,1])
      | plot([6.5,7.5],[1,1])
      | plot([8.5,9.5],[1,1])
      | color('white');
      | plot([1,1.5],[4,4])
      | plot([2.5,3.5],[4,4])
      | plot([4.5,5.5],[4,4])
      | plot([6.5,7.5],[4,4])
      | plot([8.5,9.5],[4,4])
  Generate  limited decrease for partition1 variant2 1 : Subsystem  mask(Feature generation){X0=0.5, XF=0, T=2}
      mask prompts: X0 "Initial output:"; XF "Final output:"; T "Duration"
      mask help: Output a decreasing ramp signal limited from bottom and top, starting at the specified time.
      mask Display:
      | plot([1:10],[4,4,4,4,4,1,1,1,1,1])
      | plot([1:10],[4,4,4,1,1,1,1,1,1,1])
      | plot([1:10],[4,1,1,1,1,1,1,1,1,1])
      | plot([1:10],[4,4,4,4,4,1,1,1,1,1])
      | plot([1:10],[4,4,4,4,4,4,4,1,1,1])
      | plot([1:10],[4,4,4,4,4,4,4,4,4,1])
      | plot([1:10],[4,4,4,4,4,4,4,4,4,4])
      | color('white');
      | plot([1:10],[1,1,1,1,1,1,1,1,1,1])
      | color('black');
      | plot([1,1.5],[1,1])
      | plot([2.5,3.5],[1,1])
      | plot([4.5,5.5],[1,1])
      | plot([6.5,7.5],[1,1])
      | plot([8.5,9.5],[1,1])
      | color('white');
      | plot([1,1.5],[4,4])
      | plot([2.5,3.5],[4,4])
      | plot([4.5,5.5],[4,4])
      | plot([6.5,7.5],[4,4])
      | plot([8.5,9.5],[4,4])
  TestDataVariants Sequence : Subsystem
  switch : MultiPortSwitch  Inputs=2  OutDataType=sfix(16)  OutScaling=2^0
  phi_Acc : Outport  OutDataType=sfix(16)  OutScaling=2^0
  wires:
  switch/1 -> phi_Acc/1
  Generate  limited decrease for partition1 variant2 1/1(Out1) -> switch/3
  Generate  limited decrease for partition1 variant1 1/1(Out1) -> switch/2
  TestDataVariants Sequence/1(Out1) -> switch/1

== system Pedal_Interpretation_exe_gr/Test Data for PI/SR-PI-01.3 Acceleration Pedal recognition/phi_Acc >= ped_min/Generate increase 2 ==
  Generate  limited increase for partition1 variant1 1 : Subsystem  mask(Feature generation){X0=5, XF=14.5, T=2}
      mask prompts: X0 "Initial output:"; XF "Final output:"; T "Duration:"
      mask help: Output a ramp signal limited from bottom and top, starting at the specified time.
      mask Display:
      | plot([1:10],[1,1,1,1,1,4,4,4,4,4])
      | plot([1:10],[1,4,4,4,4,4,4,4,4,4])
      | plot([1:10],[1,1,1,4,4,4,4,4,4,4])
      | plot([1:10],[1,1,1,1,1,4,4,4,4,4])
      | plot([1:10],[1,1,1,1,1,1,1,4,4,4])
      | plot([1:10],[1,1,1,1,1,1,1,1,1,4])
      | plot([5:10],[1,1,1,1,1,1])
      | color('white');
      | plot([1:10],[4,4,4,4,4,4,4,4,4,4])
      | color('white');
      | plot([1,1.5],[1,1])
      | plot([2.5,3.5],[1,1])
      | plot([4.5,5.5],[1,1])
      | plot([6.5,7.5],[1,1])
      | plot([8.5,9.5],[1,1])
      | color('black');
      | plot([1,1.5],[4,4])
      | plot([2.5,3.5],[4,4])
      | plot([4.5,5.5],[4,4])
      | plot([6.5,7.5],[4,4])
      | plot([8.5,9.5],[4,4])
  Generate  limited increase for partition1 variant2 1 : Subsystem  mask(Feature generation){X0=90.5, XF=100, T=2}
      mask prompts: X0 "Initial output:"; XF "Final output:"; T "Duration:"
      mask help: Output a ramp signal limited from bottom and top, starting at the specified time.
      mask Display:
      | plot([1:10],[1,1,1,1,1,4,4,4,4,4])
      | plot([1:10],[1,4,4,4,4,4,4,4,4,4])
      | plot([1:10],[1,1,1,4,4,4,4,4,4,4])
      | plot([1:10],[1,1,1,1,1,4,4,4,4,4])
      | plot([1:10],[1,1,1,1,1,1,1,4,4,4])
      | plot([1:10],[1,1,1,1,1,1,1,1,1,4])
      | plot([5:10],[1,1,1,1,1,1])
      | color('white');
      | plot([1:10],[4,4,4,4,4,4,4,4,4,4])
      | color('white');
      | plot([1,1.5],[1,1])
      | plot([2.5,3.5],[1,1])
      | plot([4.5,5.5],[1,1])
      | plot([6.5,7.5],[1,1])
      | plot([8.5,9.5],[1,1])
      | color('black');
      | plot([1,1.5],[4,4])
      | plot([2.5,3.5],[4,4])
      | plot([4.5,5.5],[4,4])
      | plot([6.5,7.5],[4,4])
      | plot([8.5,9.5],[4,4])
  TestDataVariants Sequence : Subsystem
  switch : MultiPortSwitch  Inputs=2  OutDataType=sfix(16)  OutScaling=2^0
  phi_Acc : Outport  OutDataType=sfix(16)  OutScaling=2^0
  wires:
  switch/1 -> phi_Acc/1
  Generate  limited increase for partition1 variant2 1/1(Out1) -> switch/3
  Generate  limited increase for partition1 variant1 1/1(Out1) -> switch/2
  TestDataVariants Sequence/1(Out1) -> switch/1

== system Pedal_Interpretation_exe_gr/Test Data for PI/SR-PI-02.2 Acceleration pedal interpretation/v = const & phi_Acc = const/Generate constant 5 ==
  Generate  constant for partition1 variant1 1 : Subsystem  mask(Feature generation){X0=-10, T=2}
      mask prompts: X0 "Constant value:"; T "Duration"
      mask help: Output a decreasing ramp signal limited from bottom and top, starting at the specified time.
      mask Display: plot([1:2],[4,4])
  Generate  constant for partition1 variant2 1 : Subsystem  mask(Feature generation){X0=70, T=2}
      mask prompts: X0 "Constant value:"; T "Duration"
      mask help: Output a decreasing ramp signal limited from bottom and top, starting at the specified time.
      mask Display: plot([1:2],[4,4])
  Generate  constant for partition1 variant3 1 : Subsystem  mask(Feature generation){X0=0, T=2}
      mask prompts: X0 "Constant value:"; T "Duration"
      mask help: Output a decreasing ramp signal limited from bottom and top, starting at the specified time.
      mask Display: plot([1:2],[4,4])
  Generate  constant for partition1 variant4 1 : Subsystem  mask(Feature generation){X0=-5, T=2}
      mask prompts: X0 "Constant value:"; T "Duration"
      mask help: Output a decreasing ramp signal limited from bottom and top, starting at the specified time.
      mask Display: plot([1:2],[4,4])
  Generate  constant for partition1 variant5 1 : Subsystem  mask(Feature generation){X0=35, T=2}
      mask prompts: X0 "Constant value:"; T "Duration"
      mask help: Output a decreasing ramp signal limited from bottom and top, starting at the specified time.
      mask Display: plot([1:2],[4,4])
  TestDataVariants Sequence : Subsystem
  switch : MultiPortSwitch  Inputs=5  OutDataType=sfix(16)  OutScaling=2^0
  v_Fzg : Outport  OutDataType=sfix(16)  OutScaling=2^0
  wires:
  switch/1 -> v_Fzg/1
  Generate  constant for partition1 variant2 1/1(Out1) -> switch/3
  Generate  constant for partition1 variant1 1/1(Out1) -> switch/2
  Generate  constant for partition1 variant3 1/1(Out1) -> switch/4
  Generate  constant for partition1 variant4 1/1(Out1) -> switch/5
  Generate  constant for partition1 variant5 1/1(Out1) -> switch/6
  TestDataVariants Sequence/1(Out1) -> switch/1
